simulink library "MinSegLibrary_MinSegPro"  (R2015a)
settings: Solver=ode45  StartTime=0.0  StopTime=10.0  RelTol=1e-3
libraries: arduinolib x4
settings Model: Creator=hurstj  LastModifiedBy=hurstj
settings DebuggingCC: UnderspecifiedInitializationDetection=Classic  MergeDetectMultiDrivingBlocksExec=none  SolverPrmCheckMsg=warning  StateNameClashWarn=warning

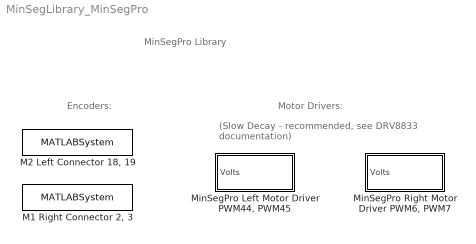
== system MinSegLibrary_MinSegPro ==
  note: (Slow Decay - recommended, see DRV8833 documentation)
  note: Motor Drivers:
  note: Encoders:
  note: MinSegPro Library
  "M1 Right Connector 2, 3" : MATLABSystem  System=Encoder_arduino  Encoder=0  PinA=2  PinB=3  PWMFSelect=3  PWMTimer=-1
      mask Type: Encoder_arduino
      mask Display:
      | disp('soEncoder');
      | port_label('output',1,'y');
  "M2 Left Connector 18, 19" : MATLABSystem  System=Encoder_arduino  Encoder=1  PinA=19  PinB=18  PWMFSelect=3  PWMTimer=-1
      mask Type: Encoder_arduino
      mask Display:
      | disp('soEncoder');
      | port_label('output',1,'y');
  "MinSegPro Left Motor Driver PWM44, PWM45" : Subsystem  mask{Vsupply=3.9, PWMoffset=0}
      mask prompts: Vsupply "Driver Voltage"; PWMoffset "PWM offset (0-255)"
      mask help:
      | Specify driver supply voltage (3.9 for USB)
      | Specify the PWM offset (0-255)
      mask Display:
      | port_label('input',1,'Volts')
      | text(15,5,['Vsupply=' num2str(Vsupply)])
  "MinSegPro Right Motor Driver PWM6, PWM7 " : Subsystem  mask{Vsupply=3.9, PWMoffset=0}
      mask prompts: Vsupply "Driver Voltage"; PWMoffset "PWM offset (0-255)"
      mask help:
      | Specify driver supply voltage (3.9 for USB)
      | Specify the PWM offset (0-255)
      mask Display:
      | port_label('input',1,'Volts')
      | text(15,5,['Vsupply=' num2str(Vsupply)])

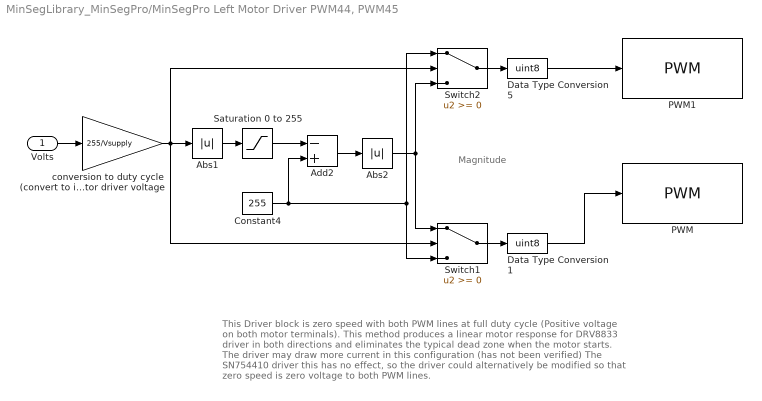
== system MinSegLibrary_MinSegPro/MinSegPro Left Motor Driver PWM44, PWM45 ==
  note: Magnitude
  note: This Driver block is zero speed with both PWM lines at full duty cycle
      |  (Positive voltage on both motor terminals).
      | This method produces a linear motor response for DRV8833 driver
      |  in both directions and eliminates
      | the typical dead zone when the motor starts.
      | The driver may draw more current in this configuration (has not been verified)
      |
      | The SN754410 driver this has no effect, so the driver could alternatively
      | be modified so that zero speed is zero voltage to both PWM lines.
  Volts : Inport
  Abs1 : Abs
  Abs2 : Abs
  Add2 : Sum  Inputs=-+
  Constant4 : Constant  Value=255
  Data Type Conversion1 : DataTypeConversion  OutDataTypeStr=uint8
  Data Type Conversion5 : DataTypeConversion  OutDataTypeStr=uint8
  PWM : arduinolib/PWM  pinNumber=45  blockPlatform=arduino
  PWM1 : arduinolib/PWM  pinNumber=44  blockPlatform=arduino
  Saturation 0 to 255 : Saturate  UpperLimit=255  LowerLimit=0
  Switch1 : Switch
  Switch2 : Switch
  conversion to duty cycle (convert to int) denominator is motor driver voltage : Gain  Gain=255/Vsupply  OutDataTypeStr=int16
  wires:
  Data Type Conversion1/1 -> PWM/1
  Data Type Conversion5/1 -> PWM1/1
  Switch1/1 -> Data Type Conversion1/1
  Switch2/1 -> Data Type Conversion5/1
  Abs2/1 -> Switch1/1, Switch2/3
  Add2/1 -> Abs2/1
  Constant4/1 -> Add2/2, Switch2/1, Switch1/3
  Abs1/1 -> Saturation 0 to 255/1
  Saturation 0 to 255/1 -> Add2/1
  conversion to duty cycle (convert to int) denominator is motor driver voltage/1 -> Switch1/2, Abs1/1, Switch2/2
  Volts/1 -> conversion to duty cycle (convert to int) denominator is motor driver voltage/1

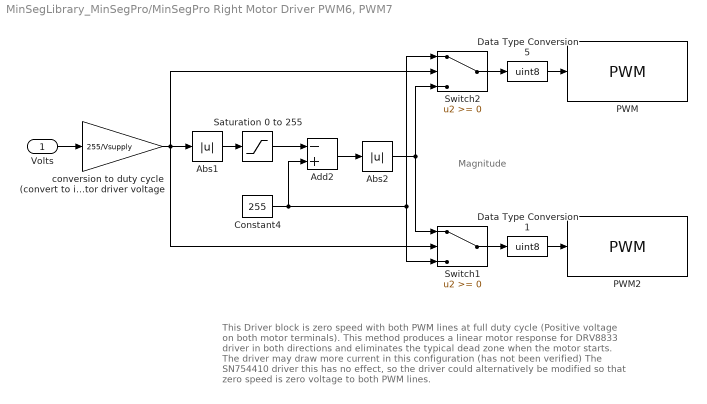
== system MinSegLibrary_MinSegPro/MinSegPro Right Motor Driver PWM6, PWM7  ==
  note: Magnitude
  note: This Driver block is zero speed with both PWM lines at full duty cycle
      |  (Positive voltage on both motor terminals).
      | This method produces a linear motor response for DRV8833 driver
      |  in both directions and eliminates
      | the typical dead zone when the motor starts.
      | The driver may draw more current in this configuration (has not been verified)
      |
      | The SN754410 driver this has no effect, so the driver could alternatively
      | be modified so that zero speed is zero voltage to both PWM lines.
  Volts : Inport
  Abs1 : Abs
  Abs2 : Abs
  Add2 : Sum  Inputs=-+
  Constant4 : Constant  Value=255
  Data Type Conversion1 : DataTypeConversion  OutDataTypeStr=uint8
  Data Type Conversion5 : DataTypeConversion  OutDataTypeStr=uint8
  PWM : arduinolib/PWM  pinNumber=6  blockPlatform=arduino
  PWM2 : arduinolib/PWM  pinNumber=7  blockPlatform=arduino
  Saturation 0 to 255 : Saturate  UpperLimit=255  LowerLimit=0
  Switch1 : Switch
  Switch2 : Switch
  conversion to duty cycle (convert to int) denominator is motor driver voltage : Gain  Gain=255/Vsupply  OutDataTypeStr=int16
  wires:
  Data Type Conversion1/1 -> PWM2/1
  Data Type Conversion5/1 -> PWM/1
  Switch1/1 -> Data Type Conversion1/1
  Switch2/1 -> Data Type Conversion5/1
  Abs2/1 -> Switch1/1, Switch2/3
  Add2/1 -> Abs2/1
  Constant4/1 -> Add2/2, Switch2/1, Switch1/3
  Abs1/1 -> Saturation 0 to 255/1
  Saturation 0 to 255/1 -> Add2/1
  conversion to duty cycle (convert to int) denominator is motor driver voltage/1 -> Switch1/2, Switch2/2, Abs1/1
  Volts/1 -> conversion to duty cycle (convert to int) denominator is motor driver voltage/1
